simulink model "Task_6_template"  (R2023b)
settings: Solver=FixedStepDiscrete  StartTime=0.0  StopTime=t_all(end)  FixedStep=0.01  RelTol=1e-3
PreLoadFcn:
  | load init_values_task2.mat
settings Model: DataTypeOverride=Off  FPTShortcutValueString='{{},{''BaselineRun_2'',1,1,1,''BaselineRun_2'','''',{},''M'','''',''''}}'  PauseTimes=1  Creator=Mateusz  LastModifiedBy=kacper
settings OptimizationCC: BlockReduction=off  ConditionallyExecuteInputs=off  DefaultParameterBehavior=Inlined  InheritOutputTypeSmallerThanSingle=on
settings DebuggingCC: SignalRangeChecking=warning  AlgebraicLoopMsg=error  SingleTaskRateTransMsg=error
settings HardwareCC: ProdBitPerPointer=32  ProdBitPerSizeT=32  ProdBitPerPtrDiffT=32  ProdLargestAtomicFloat=None  ProdIntDivRoundTo=Undefined  ProdEndianess=Unspecified  ProdWordSize=32  ProdHWDeviceType=ASIC/FPGA->ASIC/FPGA  TargetBitPerLong=64  TargetBitPerPointer=64  TargetBitPerSizeT=64  TargetBitPerPtrDiffT=64  TargetLongLongMode=on  TargetIntDivRoundTo=Zero  TargetEndianess=LittleEndian  TargetWordSize=64  TargetHWDeviceType=Custom Processor->MATLAB Host Computer  ProdEqTarget=off

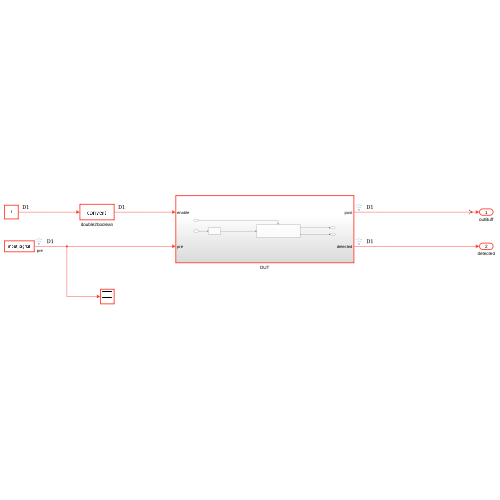
[thumbnail: Simulink's stored preview of the top-level diagram]
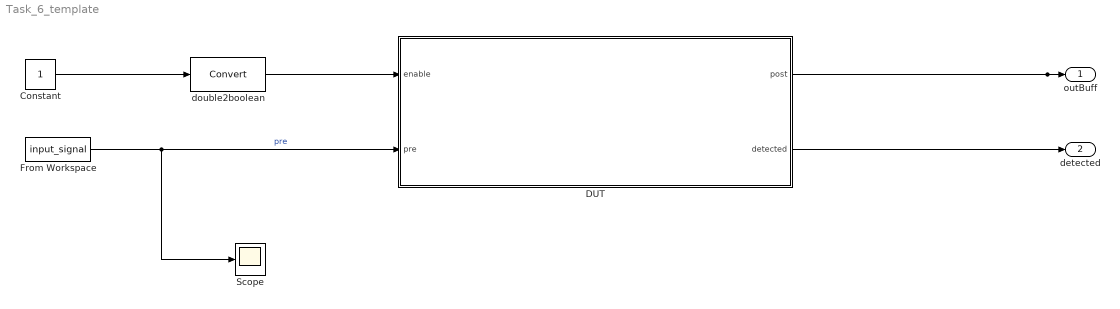
== system Task_6_template ==
  Constant : Constant  SampleTime=0.01
  DUT : Subsystem
  From Workspace : FromWorkspace  VariableName=input_signal  SampleTime=0.01
  Scope : Scope
  double2boolean : DataTypeConversion  SaturateOnIntegerOverflow=off  RndMeth=Floor
  outBuff : Outport
  detected : Outport  Port=2
  wires:
  From Workspace/1 -> Scope/1, DUT/2(pre)  "pre"
  DUT/2(detected) -> detected/1
  DUT/1(post) -> outBuff/1
  Constant/1 -> double2boolean/1
  double2boolean/1 -> DUT/1(enable)

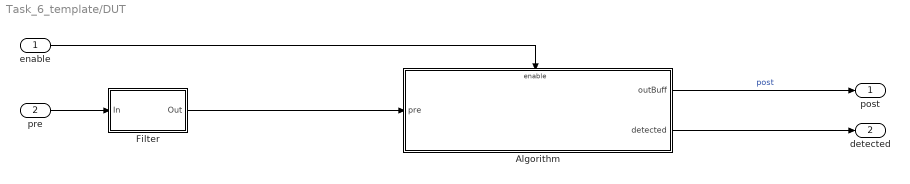
== system Task_6_template/DUT ==
  enable : Inport  OutDataTypeStr=boolean
  pre : Inport  Port=2
  Algorithm : Subsystem
  Filter : Subsystem  Tag=BlockMethodSubSystem
  post : Outport  OutDataTypeStr=int8
  detected : Outport  Port=2  OutDataTypeStr=boolean
  wires:
  Algorithm/1(outBuff) -> post/1  "post"
  Algorithm/2(detected) -> detected/1
  pre/1 -> Filter/1(In)
  enable/1 -> Algorithm/Enable
  Filter/1(Out) -> Algorithm/1(pre)

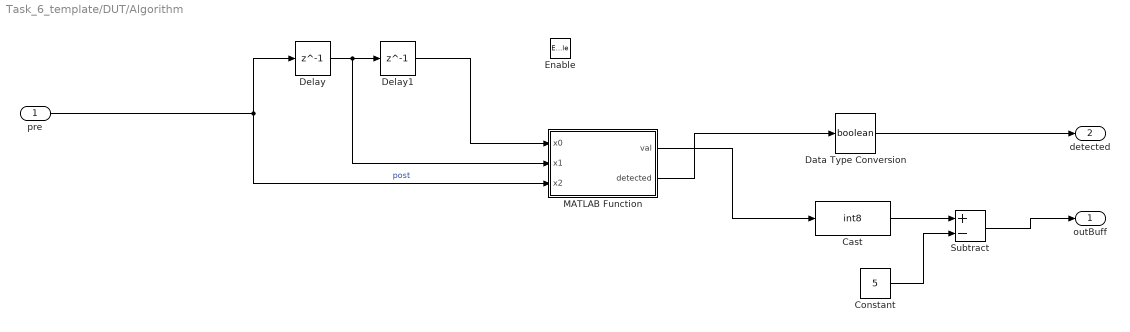
== system Task_6_template/DUT/Algorithm ==
  pre : Inport
  Enable : EnablePort
  Cast : DataTypeConversion  OutDataTypeStr=int8  SaturateOnIntegerOverflow=off  RndMeth=Floor
  Constant : Constant  Value=5  OutDataTypeStr=int8  SampleTime=-1
  Data Type Conversion : DataTypeConversion  OutDataTypeStr=boolean  RndMeth=Nearest  SaturateOnIntegerOverflow=off
  Delay : Delay  DelayLength=1
  Delay1 : Delay  DelayLength=1
  MATLAB Function : MATLAB Function  TreatAsAtomicUnit=on
  Subtract : Sum  Inputs=+-  OutDataTypeStr=int8
  outBuff : Outport  InitialOutput=0
  detected : Outport  Port=2  InitialOutput=0
  wires:
  Delay/1 -> MATLAB Function/2(x1), Delay1/1
  pre/1 -> MATLAB Function/3(x2), Delay/1  "post"
  Delay1/1 -> MATLAB Function/1(x0)
  Data Type Conversion/1 -> detected/1
  Cast/1 -> Subtract/1
  Subtract/1 -> outBuff/1
  Constant/1 -> Subtract/2
  MATLAB Function/1(val) -> Cast/1
  MATLAB Function/2(detected) -> Data Type Conversion/1

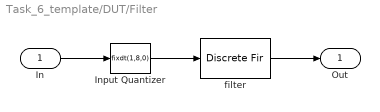
== system Task_6_template/DUT/Filter ==
  In : Inport
  Input Quantizer : DataTypeConversion  OutDataTypeStr=fixdt(1,8,0)  RndMeth=Round
  filter : DiscreteFir  Coefficients=[-0.0380175017460085002 -0.00322567352420052638 0.0669934112770634305 0.153739668396551454 0.225568942069223038 0.253428644008794834 0.225568942069223038 0.153739668396551454 0.0669934112770634305 -0.00322567352420052638 -0.0380175017460085002]  InputProcessing=Columns as channels (frame based)  CoefDataTypeStr=fixdt(true,16,16)  ProductDataTypeStr=fixdt(true,23,16)  AccumDataTypeStr=fixdt(true,25,16)  OutDataTypeStr=fixdt(true,25,16)  RndMeth=Convergent
  Out : Outport
  wires:
  In/1 -> Input Quantizer/1
  Input Quantizer/1 -> filter/1
  filter/1 -> Out/1

== matlab function Task_6_template/DUT/Algorithm/MATLAB Function ==
  data: x0 input; val output; x1 input; x2 input; detected output
function [val, detected] = fcn(x0, x1, x2)
    detected = boolean(false);
    val = int8(0);
    u   = int8(0);

    
    if x1 > x2 && x1 > x0 
        u = int8(x1);
        detected = true;
    else
        detected = false;
    end
    
val = int8(u);
detected = detected;
